simulink library "pingui"  (R2025a)
settings: Solver=VariableStepAuto  StartTime=0.0  StopTime=10.0  RelTol=1e-3
libraries: etargetslib x5
settings Model: Creator=damerius  LastModifiedBy=damerius

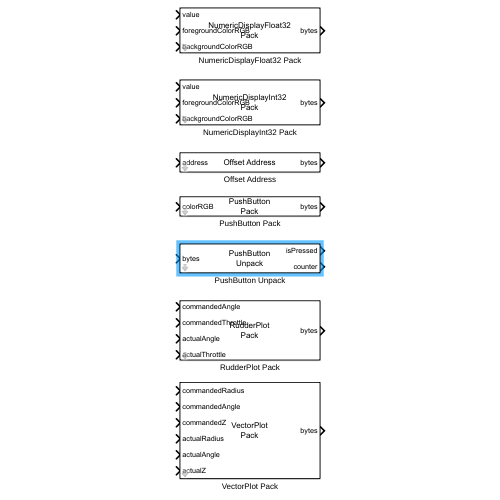
[thumbnail: Simulink's stored preview of the top-level diagram]
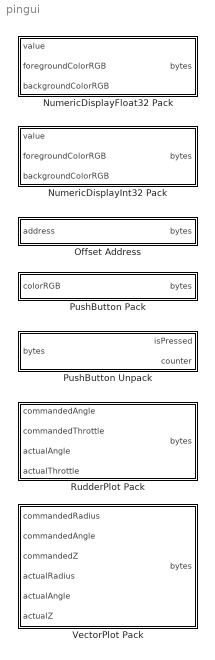
== system pingui ==
  NumericDisplayFloat32 Pack : Subsystem
      mask help: Pack a message for the NumericDisplayFloat32 widget.
      mask DialogControl DescGroupVar Prompt: NumericDisplayFloat32 Pack
      mask Display: disp('NumericDisplayFloat32\nPack');
  NumericDisplayInt32 Pack : Subsystem
      mask help: Pack a message for the NumericDisplayInt32 widget.
      mask DialogControl DescGroupVar Prompt: NumericDisplayInt32 Pack
      mask Display: disp('NumericDisplayInt32\nPack');
  Offset Address : Subsystem
      mask help: Pack the offset address to be send to the pingui application.
      mask DialogControl DescGroupVar Prompt: Offset Address
      mask Display: disp('Offset Address');
  PushButton Pack : Subsystem
      mask help: Pack a message for the PushButton widget.
      mask DialogControl DescGroupVar Prompt: PushButton Pack
      mask Display: disp('PushButton\nPack');
  PushButton Unpack : Subsystem
      mask help: Unpack a message from the PushButton widget.
      mask DialogControl DescGroupVar Prompt: PushButton Unpack
      mask Display: disp('PushButton\nUnpack');
  RudderPlot Pack : Subsystem
      mask help: Pack a message for the RudderPlot widget.
      mask DialogControl DescGroupVar Prompt: RudderPlot Pack
      mask Display: disp('RudderPlot\nPack');
  VectorPlot Pack : Subsystem
      mask help: Pack a message for the VectorPlot widget.
      mask DialogControl DescGroupVar Prompt: VectorPlot Pack
      mask Display: disp('VectorPlot\nPack');

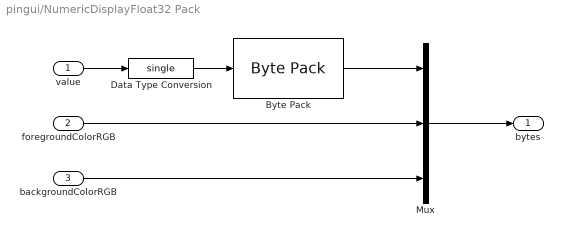
== system pingui/NumericDisplayFloat32 Pack ==
  value : Inport  PortDimensions=1
  foregroundColorRGB : Inport  Port=2  OutDataTypeStr=uint8  PortDimensions=3
  backgroundColorRGB : Inport  Port=3  OutDataTypeStr=uint8  PortDimensions=3
  Byte Pack : etargetslib/Byte Pack  datatypes={'single'}  byteAlign=1
  Data Type Conversion : DataTypeConversion  OutDataTypeStr=single  SaturateOnIntegerOverflow=off  RndMeth=Floor
  Mux : Mux  Inputs=3
  bytes : Outport
  wires:
  Byte Pack/1 -> Mux/1
  Mux/1 -> bytes/1
  backgroundColorRGB/1 -> Mux/3
  foregroundColorRGB/1 -> Mux/2
  value/1 -> Data Type Conversion/1
  Data Type Conversion/1 -> Byte Pack/1

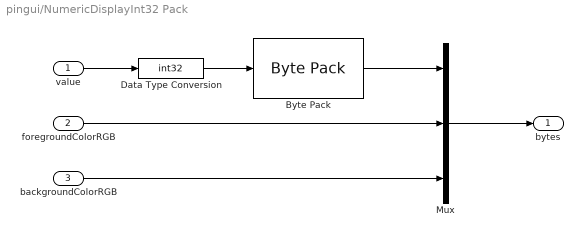
== system pingui/NumericDisplayInt32 Pack ==
  value : Inport  PortDimensions=1
  foregroundColorRGB : Inport  Port=2  OutDataTypeStr=uint8  PortDimensions=3
  backgroundColorRGB : Inport  Port=3  OutDataTypeStr=uint8  PortDimensions=3
  Byte Pack : etargetslib/Byte Pack  datatypes={'int32'}  byteAlign=1
  Data Type Conversion : DataTypeConversion  OutDataTypeStr=int32  SaturateOnIntegerOverflow=off  RndMeth=Floor
  Mux : Mux  Inputs=3
  bytes : Outport
  wires:
  value/1 -> Data Type Conversion/1
  Byte Pack/1 -> Mux/1
  foregroundColorRGB/1 -> Mux/2
  backgroundColorRGB/1 -> Mux/3
  Mux/1 -> bytes/1
  Data Type Conversion/1 -> Byte Pack/1

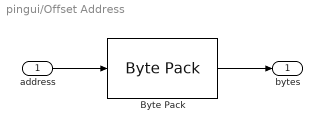
== system pingui/Offset Address ==
  address : Inport  OutDataTypeStr=uint32  PortDimensions=1
  Byte Pack : etargetslib/Byte Pack  datatypes={'uint32'}  byteAlign=1
  bytes : Outport  OutDataTypeStr=uint8  PortDimensions=4
  wires:
  address/1 -> Byte Pack/1
  Byte Pack/1 -> bytes/1

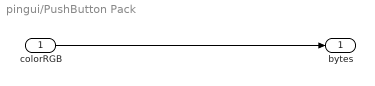
== system pingui/PushButton Pack ==
  colorRGB : Inport  OutDataTypeStr=uint8  PortDimensions=3
  bytes : Outport  OutDataTypeStr=uint8  PortDimensions=3
  wires:
  colorRGB/1 -> bytes/1

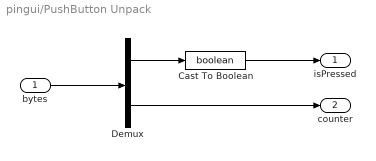
== system pingui/PushButton Unpack ==
  bytes : Inport  OutDataTypeStr=uint8  PortDimensions=2
  Cast To Boolean : DataTypeConversion  OutDataTypeStr=boolean  SaturateOnIntegerOverflow=off  RndMeth=Floor
  Demux : Demux  Outputs=2
  isPressed : Outport  OutDataTypeStr=boolean  PortDimensions=1
  counter : Outport  Port=2  OutDataTypeStr=uint8  PortDimensions=1
  wires:
  bytes/1 -> Demux/1
  Demux/1 -> Cast To Boolean/1
  Demux/2 -> counter/1
  Cast To Boolean/1 -> isPressed/1

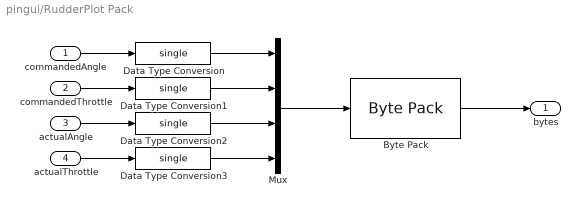
== system pingui/RudderPlot Pack ==
  commandedAngle : Inport  Unit=rad  PortDimensions=1
  commandedThrottle : Inport  Port=2  PortDimensions=1
  actualAngle : Inport  Port=3  Unit=rad  PortDimensions=1
  actualThrottle : Inport  Port=4  PortDimensions=1
  Byte Pack : etargetslib/Byte Pack  datatypes={'single'}  byteAlign=1
  Data Type Conversion{,1..3} (4 alike) : DataTypeConversion  OutDataTypeStr=single  SaturateOnIntegerOverflow=off  RndMeth=Floor
  Mux : Mux
  bytes : Outport  OutDataTypeStr=uint8  PortDimensions=16
  wires:
  commandedAngle/1 -> Data Type Conversion/1
  commandedThrottle/1 -> Data Type Conversion1/1
  actualAngle/1 -> Data Type Conversion2/1
  actualThrottle/1 -> Data Type Conversion3/1
  Data Type Conversion/1 -> Mux/1
  Data Type Conversion1/1 -> Mux/2
  Data Type Conversion2/1 -> Mux/3
  Data Type Conversion3/1 -> Mux/4
  Mux/1 -> Byte Pack/1
  Byte Pack/1 -> bytes/1

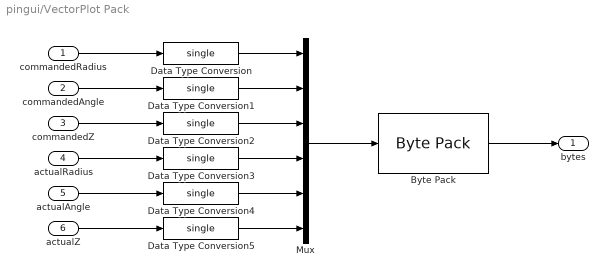
== system pingui/VectorPlot Pack ==
  commandedRadius : Inport  PortDimensions=1
  commandedAngle : Inport  Port=2  Unit=rad  PortDimensions=1
  commandedZ : Inport  Port=3  PortDimensions=1
  actualRadius : Inport  Port=4  PortDimensions=1
  actualAngle : Inport  Port=5  Unit=rad  PortDimensions=1
  actualZ : Inport  Port=6  PortDimensions=1
  Byte Pack : etargetslib/Byte Pack  datatypes={'single'}  byteAlign=1
  Data Type Conversion{,1..5} (6 alike) : DataTypeConversion  OutDataTypeStr=single  SaturateOnIntegerOverflow=off  RndMeth=Floor
  Mux : Mux  Inputs=6
  bytes : Outport  OutDataTypeStr=uint8  PortDimensions=24
  wires:
  Data Type Conversion/1 -> Mux/1
  Data Type Conversion1/1 -> Mux/2
  Data Type Conversion2/1 -> Mux/3
  Data Type Conversion3/1 -> Mux/4
  Mux/1 -> Byte Pack/1
  Data Type Conversion5/1 -> Mux/6
  Data Type Conversion4/1 -> Mux/5
  Byte Pack/1 -> bytes/1
  commandedRadius/1 -> Data Type Conversion/1
  commandedAngle/1 -> Data Type Conversion1/1
  commandedZ/1 -> Data Type Conversion2/1
  actualRadius/1 -> Data Type Conversion3/1
  actualAngle/1 -> Data Type Conversion4/1
  actualZ/1 -> Data Type Conversion5/1
